simulink model "wednesday_stuff"  (R2022b)
settings: Solver=FixedStepAuto  StartTime=0.0  StopTime=Inf  RelTol=1e-3  EnableMultiTasking=on
values from neighbouring files (symbols this model uses):
  A = [A_sub-k_c.*Bd_sub*C_sub, k_c.*Bd_sub*C_sub; k_c.*Bd_sub2*C_sub, A_sub2-k_c.*Bd_sub2*C_sub]    [doubpend.m]
  b = 0    [doubpend.m]
  J_pend = J_rotor    (= 1.911e-05)    [doubpend.m]
  K_g = m*g*l_c    (= 0.00896720076)    [doubpend.m]
  K_m = 3.9e-2    (= 0.039)    [doubpend.m]
  K_pend = 0    [doubpend.m]
  K_SF = K_aug(1:size(A_d,1))    [doubpend.m]
  K_sin = cos(Angle_Pendu)    [doubpend.m]
  L = 0.23e-3    (= 0.00023)    [doubpend.m]
  L_Pred = L_Pred'    [doubpend.m]
  N = 1/freqresp(TF_yrf,[0])    [doubpend.m]
  R = 8.985    [doubpend.m]
  Stepsize = 1    [doubpend.m]
  Ts = 0.001    [doubpend.m]
  V_s = 10.72    [doubpend.m]
undefined symbols (not defined in the file or in its folder): A_d, B_d, C_d, Down, GPTRIP1SEL, GPTRIP2SEL, TZ1, TZ2, Up
libraries: tiiqmathlib x4, c2837xDlib x1, simulink x1, embmathops x1, c2802xlib x1, c280xlib x1
settings Model: ExtModeTrigDuration=8  Creator=hanw  LastModifiedBy=pruth
settings SolverCC: AutoInsertRateTranBlk=on
settings DataIOCC: InspectSignalLogs=on
settings OptimizationCC: DefaultUnderspecifiedDataType=single  EnhancedBackFolding=on  PassReuseOutputArgsAs=Individual arguments  MaxStackSize=1024  OptimizeBlockOrder=speed  DifferentSizesBufferReuse=on  OptimizationCustomize=off  DenormalBehavior=FlushToZero  EfficientTunableParamExpr=on
settings DebuggingCC: ParameterTunabilityLossMsg=error
settings HardwareCC: ProdBitPerChar=16  ProdBitPerInt=16  ProdBitPerPointer=32  ProdBitPerSizeT=32  ProdBitPerPtrDiffT=32  ProdLargestAtomicInteger=Integer  ProdLargestAtomicFloat=None  ProdWordSize=16  ProdLongLongMode=on  ProdHWDeviceType=Texas Instruments->C2000
settings ModelReferenceCC: ModelReferenceNumInstancesAllowed=Single
settings SFSimCC: MATLABDynamicMemAlloc=off
settings RTWCC: Description=Embedded Coder  SystemTargetFile=ert.tlc  HardwareBoard=TI Delfino F28379D LaunchPad  TLCOptions=-aInlineSetEventsForThisBaseRateFcn=TLC_FALSE -aSuppressMultiTaskScheduler=TLC_FALSE -aRateBasedStepFcn=1  TemplateMakefile=ert_default_tmf  Toolchain=Texas Instruments Code Composer Studio (C2000)
settings CodeAppCC: ForceParamTrailComments=on  IgnoreCustomStorageClasses=off  OperatorAnnotations=on  SimulinkDataObjDesc=on  SFDataObjDesc=on  InsertBlockDesc=on
settings ERTTargetCC: CodeReplacementLibrary=TI C28x  ExtModeTransport=4  ExtModeStaticAlloc=on  ExtModeMexFile=ext_xcp  ExtModeIntrfLevel=Level2 - Open

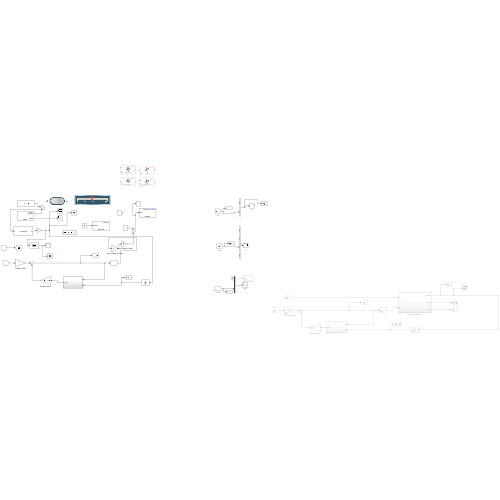
[thumbnail: Simulink's stored preview of the top-level diagram]
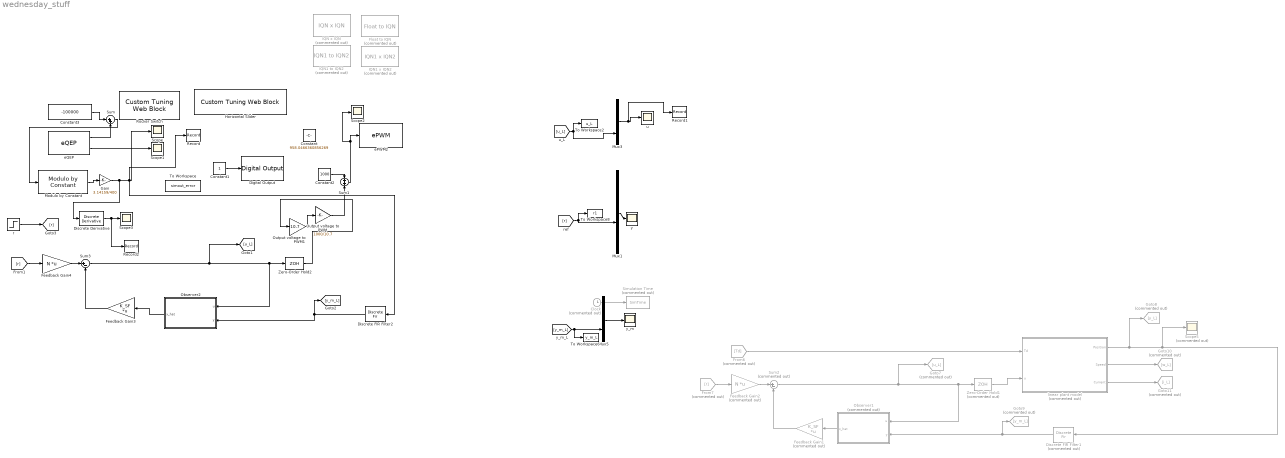
== system wednesday_stuff ==
  Clock : Clock  Commented=on
  Constant : Constant  Value=958.0466360856269
  Constant1 : Constant
  Constant2 : Constant  Value=1000
  Constant3 : Constant  Value=-100000
  Digital Output : c2837xDlib/Digital Output  GPIO_Number=GPIO0~GPIO7  GPIO_Bit0=off  GPIO_BIT0_Toggle=off  GPIO_Bit1=off  GPIO_BIT1_Toggle=off  GPIO_Bit2=on  GPIO_BIT2_Toggle=off  GPIO_Bit3=off  GPIO_BIT3_Toggle=off  GPIO_Bit4=off  GPIO_BIT4_Toggle=off  GPIO_Bit5=off  GPIO_BIT5_Toggle=off  GPIO_Bit6=off  GPIO_BIT6_Toggle=off  GPIO_Bit7=off  GPIO_BIT7_Toggle=off
  Discrete Derivative : simulink/Discrete/Discrete Derivative  gainval=1.0  ICPrevScaledInput=0.0  OutMin=[]  OutMax=[]  OutDataType=fixdt(1, 16)  OutScaling=2^-10  DoSatur=off
  Discrete FIR Filter1 : DiscreteFir  Commented=on  Coefficients=[1]  SampleTime=Ts
  Discrete FIR Filter2 : DiscreteFir  Coefficients=[1]  SampleTime=Ts
  Feedback Gain1 : Gain  Commented=on  Gain=K_SF  Multiplication=Matrix(K*u)
  Feedback Gain2 : Gain  Commented=on  Gain=N  Multiplication=Matrix(K*u)
  Feedback Gain3 : Gain  Gain=K_SF  Multiplication=Matrix(K*u)
  Feedback Gain4 : Gain  Gain=N  Multiplication=Matrix(K*u)
  Float to IQN : tiiqmathlib/Float to IQN  Commented=on  Q_value=10
  From6 : From  Commented=on  GotoTag=Td
  From7 : From  Commented=on  GotoTag=r
  Gain : Gain  Gain=3.14159/400
  Goto10 : Goto  Commented=on  GotoTag=w_L
  Goto11 : Goto  Commented=on  GotoTag=i_L
  Goto7 : Goto  Commented=on  GotoTag=u_L
  Goto8 : Goto  Commented=on  GotoTag=y_L
  Goto9 : Goto  Commented=on  GotoTag=y_m_L
  Horizontal Slider : CustomTuningWebBlock  LabelPosition=Hide  ShowInitialText=on  Configuration="{\"components\":[{\"name\":\"LinearScaleComponent\",\"settings\":{\"bounds\":{\"max\":2000,\"min\":0,\"tickInterval\":\"auto\"},\"internalTickHeightScaleFactor\":0.5,\"labelColor\":[255,255,200],\"labelFont\":{\"font\":\"Arial\",\"fontSize\":12},\"labelOffset\":0.05,\"labelTransparency\":1,\"needleImage\":{\"size\":[596,842],\"src\":\"data:image\\/svg+xml;base64,PD94bWwgdmVyc2lvbj0iMS4wIiBlbmNvZGluZz0idXRmLTgiPz4NCjwhLS0gR2VuZXJhdG9yOiBBZG9iZSBJbGx1c3RyYXRvciAyNS4wLjAsIFNWRyBFeHBvcnQgUGx1Zy1JbiAuIFNWRyBWZXJzaW9uOiA2LjAwIEJ1aWxkIDApICAtLT4NCjxzdmcgdmVyc2lvbj0iMS4xIg0KCSBpZD0ic3ZnOCIgeG1sbnM6Y2M9Imh0dHA6Ly9jcmVhdGl2ZWNvbW1vbnMub3JnL25zIyIgeG1sbnM6ZGM9Imh0dHA6Ly9wdXJsLm9yZy9kYy9lbGVtZW50cy8xLjEvIiB4bWxuczppbmtzY2FwZT0iaHR0cDovL3d3dy5pbmtzY2FwZS5vcmcvbmFtZXNw ...(+2420 chars)\",\"srcOrientation\":\"Right\"},\"needleOffset\":[-0.8044596912521441,-0.0642123287671233],\"needleSize\":{\"height\":0.4337797619047619,\"width\":0.07668067226890757},\"position\":[0.2829861111111111,0.04398634453781513,0.9196428571428571,0.6088789682539683],\"referencePoint\":\"auto\",\"scaleColors\":[],\"scaleColorsSize\":0.2,\"scaleDirection\":\"LR\",\"showLabels\":1,\"showMinorTicks\":0,\"showSpanLine\":1,\"showTicks\":1,\"tickColor\":[252,252,197],\"tickTransparency\":1,\"valueBarColor\":[0,114,189],\"valueBarOffset\":-0.27,\"valueBarSize\":0.1,\"valueBarTransparency\":1}},{\"name\":\"BackgroundImageComponent\",\"settings\":{\"image\":{\"size\":[380,101],\"src\":\"data:image\\/svg+xml;base64,PHN2ZyB4bWxucz0iaHR0cDovL3d3dy53My5vcmcvMjAwMC9zdmciIHhtbG5zOnhsaW5rPSJodHRwOi8vd3d3LnczLm9yZy8xOTk5L3hsaW5rIiB2aWV3Qm94PSIwIDAgMzgwIDEwMSI+PGRlZnM+PHN0eWxlPi5jbHMtMXtmaWxsOiMwMDJiNDI7fS5jbHMtMntmaWxsOiM0MjcwODI7fS5jbHMtM3tmaWxsOnVybCgjcmFkaWFsLWdyYWRpZW50KTt9LmNscy00e2ZpbGw6I2M4YzhjODtzdHJva2U6IzAwMDt9PC9zdHlsZT48cmFkaWFsR3JhZGllbnQgaWQ9InJhZGlhbC1ncmFkaWVudCIgY3g9IjE5MCIgY3k9IjUwLjUiIHI9IjI2OS4yMSIgZ3JhZGllbnRVbml0cz0idXNlclNwYWNlT25Vc2UiPjxzdG9wIG9mZnNldD0iMC4wMSIgc3RvcC1jb2xvcj0iIzNlNGY1OCIvPjxzdG9wIG9mZnNldD0iMC4wNiIgc3RvcC1jb2xvcj0iIzQ0NTc2MSIvPjxzdG9wIG9mZnNldD0iMC4xNSIgc3RvcC1jb2xvcj0iIzU1NmE3NiIvPjxzdG9wIG9mZnNldD0iMC4yNSIgc3RvcC1jb2xvcj0iIzZkODg5NSIvPjxzdG9wIG9mZnNldD0iMC4zOCIgc3RvcC1jb2xvcj0iIzhmYjJjMyIvPjxzdG9wIG9mZnNldD0iMC41MiIgc3RvcC1jb2xvcj0iI2I2ZTRmYSIvPjxzdG9wIG9mZnNldD0iMSIgc3RvcC1jb2xvcj0iIzE1NDY1NyIvPjwvcmFkaWFsR3JhZGllbnQ+PC9kZWZzPjxnIGlkPSJmcmFtZSI+PGcgaWQ9IkxheWVyXzIiIGRhdGEtbmFtZT0iTGF5ZXIgMiI+PGcgaWQ9IkxheWVyXzEtMiIgZGF0YS1uYW1lPSJMYXllciAxLTIiPjxyZWN0IGlkPSJyZWN0MTAzNiIgY2xhc3M9ImNscy0xIiB4PSIxMSIgeT0iMTEiIHdpZHRoPSIzNTgiIGhlaWdodD0iNzkiLz48cGF0aCBpZD0icGF0aDEwMzgiIGNsYXNzPSJjbHMtMiIgZD0iTTgsOFY5M0gzNzJWOFpNMzY5LDkwSDExVjExSDM2OVoiLz48cGF0aCBpZD0icGF0aDEwNDAiIGNsYXNzPSJjbHMtMyIgZD0iTTAsMFYxMDFIMzgwVjBaTTM3Miw5M0g4VjhIMzcyWiIvPjwvZz48L2c+PC9nPjxnIGlkPSJ0cmFjayI+PHBhdGggaWQ9InJlY3QxNjExIiBjbGFzcz0iY2xzLTQiIGQ9Ik0zMy4zNywyNi41OUgzNDYuNjNjNCwwLDcuMjUsMi42LDcuMjUsNS44MWgwYzAsMy4yMS0zLjI1LDUuODItNy4yNSw1LjgySDMzLjM3Yy00LDAtNy4yNS0yLjYxLTcuMjUtNS44MmgwQzI2LjEyLDI5LjE5LDI5LjM3LDI2LjU5LDMzLjM3LDI2LjU5WiIvPjwvZz48L3N2Zz4=\",\"srcOrientation\":\"horizontal\"},\"position\":[0,0,1,1],\"scaleMode\":\"0\"}},{\"name\":\"ForegroundImageComponent\",\"settings\":{\"image\":{\"size\":[0,0],\"src\":\"default\",\"srcOrientation\":[]},\"isForeground\":1,\"position\":[0,0,1,1],\"scaleMode\":\"0\"}}],\"settings\":{\"BindingType\":\"param\",\"aspectRatio\":3.7777777777777777,\"backgroundColor\":[0,0,0,\"1\"],\"backgroundOffset\":0,\"backgroundOpacity\":1,\"fixedAspectRatio\":\"on\",\"foregroundColor\":[252,252,196],\"orientation\":\"horizontal\",\"showBackgroundColor\":false,\"value\":0,\"version\":\"R2022b\"},\"type\":\"LinearGauge\"}"
  IQN x IQN : tiiqmathlib/IQN x IQN  Commented=on  multiplyOption=Multiply
  IQN1 to IQN2 : tiiqmathlib/IQN1 to IQN2  Commented=on  New_Q=10
  IQN1 x IQN2 : tiiqmathlib/IQN1 x IQN2  Commented=on  Q=10
  Modulo by Constant : embmathops/Modulo by Constant  Denominator=400  SimulateUsing=Code generation
      settings: LibrarySourceBlock=embeddedMathLib/Modulo by Constant
  Mux1 : Mux
  Mux3 : Mux  Inputs=2
  Mux5 : Mux  Inputs=2
  Observer1 : Subsystem  Commented=on
  Observer2 : Subsystem
  Output voltage to PWM : Gain  Gain=1000/10.7
  Output voltage to PWM1 : Gain  Gain=10.7
  Record : Record  FileSettingsInternal="{\"entries\":[{\"content\":{\"excelSettings\":{\"content\":{},\"type\":\"Streamout.ExcelSettings\"}},\"type\":\"Streamout.FileSettingStorage\",\"uuid\":\"4d44a113-255c-4606-b9fa-687f08685d0f\"}],\"packageUris\":[\"http://schema.mathworks.com/mf0/streamout_blocks/R2020a\"],\"version\":\"1.0\"}"  SignalsInternal="{\"entries\":[{\"content\":{\"signals\":[{\"content\":{\"blockPath\":[\"wednesday_stuff/Record\"],\"channel\":[],\"dimensions\":[1,1],\"domain\":\"wednesday_stuff/Record\",\"lineColor\":\"#64d413\",\"plots\":[1],\"port\":1,\"sid\":[],\"signalID\":19992,\"signalName\":\"Gain\"},\"type\":\"RecordBlkView.Signal\",\"uuid\":\"3b113f77-257b-44e4-b3fb-c5bb5a30da61\"}]},\"type\":\"RecordBlkView.InputSignals\",\"uuid\":\"18fdf491-a986-43b1-906f-4e09ae16b740\"}],\"packageUris\":[\"http://schema.mathworks.com/mf0/streamout_blocks/R2020a\"],\"version\":\"1.0\"}"  VisualizationBindings="{\"sparklinesplugin\":{\"info\":[{\"bindingParametersList\":[],\"subplotID\":1}]}}"
  Record1 : Record  FileSettingsInternal="{\"entries\":[{\"content\":{\"excelSettings\":{\"content\":{},\"type\":\"Streamout.ExcelSettings\"}},\"type\":\"Streamout.FileSettingStorage\",\"uuid\":\"0aac1b3e-fee5-4f5d-83b4-dff1f84cc0c0\"}],\"packageUris\":[\"http://schema.mathworks.com/mf0/streamout_blocks/R2020a\"],\"version\":\"1.0\"}"  SignalsInternal="{\"entries\":[{\"content\":{\"signals\":[{\"content\":{\"blockPath\":[\"wednesday_stuff/Record1\"],\"channel\":[],\"dimensions\":[2],\"domain\":\"wednesday_stuff/Record1\",\"hasChildren\":true,\"lineColor\":\"#d95319\",\"plots\":[],\"port\":1,\"sid\":[],\"signalID\":19983,\"signalName\":\"Mux3\"},\"type\":\"RecordBlkView.Signal\",\"uuid\":\"6e082fb6-09ee-4524-a44a-0b124cfc634e\"},{\"content\":{\"blockPath\":[\"wednesday_stuff/Record1\"],\"channel\":[1],\"dimensions\":[2],\"domain\":\"wednesday_stuff/Record1\",\"lineColor\":\"#a2142f\",\"parentID\":19983,\"plots\":[1],\"port\":1,\"sid\":[],\"signalID\":19984,\"signalName\":\"Mux3\"},\"type\":\"RecordBlkView.Signal\",\"uuid\":\"8481b1b3-e8f1-429e-8ea8-884c20c8de04\"},{\"content\":{\"blockPath\":[\"wednesday_stuff/Record1\"],\"channel\":[2],\"dimensions\":[2],\"domain\":\"wednesday_stuff/Record1\",\"lineColor\":\"#ff6929\",\"parentID\":19983,\"plots\":[1],\"port\":1,\"sid\":[],\"signalID\":19985,\"signalName\":\"Mux3\"},\"type\":\"RecordBlkView.Signal\",\"uuid\":\"e82f2203-a385-483f-b916-afcb370bf19b\"}]},\"type\":\"RecordBlkView.InputSignals\",\"uuid\":\"b3968912-3d6b-4861-86d9-c36083a10435\"}],\"packageUris\":[\"http://schema.mathworks.com/mf0/streamout_blocks/R2020a\"],\"version\":\"1.0\"}"  VisualizationBindings="{\"sparklinesplugin\":{\"info\":[{\"bindingParametersList\":[],\"subplotID\":1}]}}"
  Record2 : Record  FileSettingsInternal="{\"entries\":[{\"content\":{\"excelSettings\":{\"content\":{},\"type\":\"Streamout.ExcelSettings\"}},\"type\":\"Streamout.FileSettingStorage\",\"uuid\":\"185a5fe7-9dc5-4829-8d1e-3b701eb1b41e\"}],\"packageUris\":[\"http://schema.mathworks.com/mf0/streamout_blocks/R2020a\"],\"version\":\"1.0\"}"  SignalsInternal="{\"entries\":[{\"content\":{\"signals\":[{\"content\":{\"blockPath\":[\"wednesday_stuff/Record2\"],\"channel\":[],\"dimensions\":[1,1],\"domain\":\"wednesday_stuff/Record2\",\"lineColor\":\"#77ac30\",\"plots\":[1],\"port\":1,\"sid\":[],\"signalID\":19978,\"signalName\":\"Discrete Derivative\"},\"type\":\"RecordBlkView.Signal\",\"uuid\":\"3faa6981-de14-4794-b670-d27a9092c6dd\"}]},\"type\":\"RecordBlkView.InputSignals\",\"uuid\":\"b823a2af-b6b8-4942-aa66-d3cc61a8ed73\"}],\"packageUris\":[\"http://schema.mathworks.com/mf0/streamout_blocks/R2020a\"],\"version\":\"1.0\"}"  VisualizationBindings="{\"sparklinesplugin\":{\"info\":[{\"bindingParametersList\":[],\"subplotID\":1}]}}"
  Rocker Switch : CustomTuningWebBlock  LabelPosition=Hide  ShowInitialText=on  Configuration="{\"components\":[{\"name\":\"CustomSwitchStateComponent\",\"settings\":{\"position\":[0,0,1,1],\"states\":[{\"HitRegion\":{\"position\":[0,0,0.5,1]},\"Image\":{\"position\":[0.13,0,1,0.75],\"size\":[1,0.75],\"src\":\"data:image\\/svg+xml;base64,PHN2ZyB4bWxucz0iaHR0cDovL3d3dy53My5vcmcvMjAwMC9zdmciIHhtbG5zOnhsaW5rPSJodHRwOi8vd3d3LnczLm9yZy8xOTk5L3hsaW5rIiB2aWV3Qm94PSIwIDAgNzUgMjQuOCI+PGRlZnM+PHN0eWxlPi5jbHMtMXtmaWxsOnVybCgjcmFkaWFsLWdyYWRpZW50KTt9LmNscy0ye2ZpbGw6dXJsKCNyYWRpYWwtZ3JhZGllbnQtMik7fS5jbHMtM3tzdHJva2U6I2IyMDAwMDtzdHJva2Utd2lkdGg6MC4yNXB4O2ZpbGw6dXJsKCNsaW5lYXItZ3JhZGllbnQpO30uY2xzLTR7ZmlsbDp1cmwoI2xpbmVhci1ncmFkaWVudC0yKTt9LmNs ...(+3576 chars)\",\"srcOrientation\":\"Right\"},\"Label\":{\"color\":[0.5019607843137255,0.5019607843137255,0.5019607843137255],\"icon\":{\"size\":[0,0],\"src\":[],\"srcOrientation\":\"Right\"},\"iconPlacement\":\"left\",\"opacity\":1,\"position\":[0.5,0.08],\"show\":true,\"text\":{\"content\":\"Off\",\"font\":\"Helvetica\",\"fontSize\":29.7154725}},\"Value\":0},{\"HitRegion\":{\"position\":[0,0.5,0.5,1]},\"Image\":{\"position\":[0.13,0,1,0.75],\"size\":[1,0.75],\"src\":\"data:image\\/svg+xml;base64,PHN2ZyB4bWxucz0iaHR0cDovL3d3dy53My5vcmcvMjAwMC9zdmciIHhtbG5zOnhsaW5rPSJodHRwOi8vd3d3LnczLm9yZy8xOTk5L3hsaW5rIiB2aWV3Qm94PSIwIDAgNzUgMjQuOCI+PGRlZnM+PHN0eWxlPi5jbHMtMXtmaWxsOnVybCgjcmFkaWFsLWdyYWRpZW50KTt9LmNscy0ye2ZpbGw6dXJsKCNyYWRpYWwtZ3JhZGllbnQtMik7fS5jbHMtM3tzdHJva2U6I2IyMDAwMDtzdHJva2Utd2lkdGg6MC4yNXB4O2ZpbGw6dXJsKCNsaW5lYXItZ3JhZGllbnQpO30uY2xzLTR7ZmlsbDp1cmwoI2xpbmVhci1ncmFkaWVudC0yKTt9LmNs ...(+3520 chars)\",\"srcOrientation\":\"Right\"},\"Label\":{\"color\":[0.5019607843137255,0.5019607843137255,0.5019607843137255],\"icon\":{\"size\":[0,0],\"src\":[],\"srcOrientation\":\"Right\"},\"iconPlacement\":\"left\",\"opacity\":1,\"position\":[0.5,0.92],\"show\":true,\"text\":{\"content\":\"On\",\"font\":\"Helvetica\",\"fontSize\":29.7154725}},\"Value\":1}]}},{\"name\":\"BackgroundImageComponent\",\"settings\":{\"image\":{\"size\":[155,70],\"src\":\"default\",\"srcOrientation\":\"Right\"},\"position\":[0,0,1,1],\"scaleMode\":\"0\"}},{\"name\":\"ForegroundImageComponent\",\"settings\":{\"image\":{\"size\":[0,0],\"src\":\"default\",\"srcOrientation\":[]},\"isForeground\":1,\"position\":[0,0,1,1],\"scaleMode\":\"0\"}}],\"settings\":{\"BindingType\":\"param\",\"backgroundColor\":[0,0,255,\"1\"],\"backgroundOffset\":0.14,\"fixedAspectRatio\":\"on\",\"foregroundColor\":[234,234,234],\"showBackgroundColor\":false,\"variant\":\"rocker\",\"version\":\"R2022b\"},\"type\":\"Switch\"}"
  Scope{,1..3} (4 alike) : Scope
  Scope5 : Scope  Commented=on
  Simulation Time : ToWorkspace  Commented=on  VariableName=SimTime  SampleTime=-1
  Sum : Sum  Inputs=|++
  Sum1 : Sum
  Sum2 : Sum  Commented=on  Inputs=|+-
  Sum3 : Sum  Inputs=|+-
  To Workspace : ToWorkspace  VariableName=simout_error  SaveFormat=Timeseries  SampleTime=-1
  To Workspace2 : ToWorkspace  VariableName=u_L  SampleTime=Ts
  To Workspace6 : ToWorkspace  VariableName=y_m_L  SampleTime=Ts
  To Workspace8 : ToWorkspace  VariableName=r1  SampleTime=Ts
  Zero-Order Hold1 : ZeroOrderHold  Commented=on  SampleTime=Ts
  Zero-Order Hold2 : ZeroOrderHold  SampleTime=Ts
  ePWM2 : c2802xlib/ePWM  PwmType=C2000_Type4  useModule=ePWM1  ePWMxLINKTBPRD=Not Linked  periodUnits=Clock cycles  timerSource=Specify via dialog  timerPeriod_clk=2000  timerPeriod_sec=0.0001  tbshadow=Counter equals to zero  countingMode=Up-Down  phaseActiveEnable=Disable  phaseDirection=Count down after sync  phaseActive=0  synchronizationEnable=off  dcaevt1Sync=off  dcbevt1Sync=off  synchronizationOption=Counter equals to zero (CTR=Zero)  dcbevt1SyncOut=off  dcaevt1SyncOut=off  cmpdSyncOut=off  cmpcSyncOut=off  cmpbSyncOut=off  zeroSyncOut=on  swfSyncOut=off  perSynchronizationOption=Counter equals to period (CTR=PRD)  clockPrescale=1  HSclockPrescale=1  enswap=off  ePWMxAStatus=on  ePWMxAactionLogic1=Do nothing  ePWMxAactionLogic2=Do nothing  ePWMxAactionLogic3=Clear  ePWMxAactionLogic4=Set  ePWMxAactionLogic5=Do nothing  ePWMxAactionLogic6=Do nothing  ePWMxACSFenable=off  ePWMxACSFvalue=Forcing disable  ePWMxASFreload=Zero  ePWMxBStatus=on  ePWMxBactionLogic1=Set  ePWMxBactionLogic2=Clear  ePWMxBactionLogic3=Do nothing  ePWMxBactionLogic4=Do nothing  ePWMxBactionLogic5=Clear  ePWMxBactionLogic6=Set  ePWMxBCSFenable=off  ePWMxBCSFvalue=Forcing disable  ePWMxBSFreload=Zero  ePWNxBOutWay=off  ePWMxLINKCMPA=Not Linked  CMPAUnits=Clock cycles  CMPASource=Input port  CMPAValue_per=50  CMPAValue_clk=floor(2000/2+1)  enCMPAshadow=Counter equals to zero (CTR=Zero)  ePWMxLINKCMPB=Not Linked  CMPBUnits=Clock cycles  CMPBSource=Specify via dialog  CMPBValue_per=50  CMPBValue_clk=floor(2000/2+1)  enCMPBshadow=Counter equals to zero (CTR=Zero)  ePWMxLINKCMPC=ePWM3  CMPCUnits=Clock cycles  CMPCSource=Specify via dialog  CMPCValue_per=50  CMPCValue_clk=32000  enCMPCshadow=Counter equals to zero (CTR=Zero)  ePWMxLINKCMPD=Not Linked  CMPDUnits=Clock cycles  CMPDSource=Specify via dialog  CMPDValue_per=50  CMPDValue_clk=1000  enCMPDshadow=Counter equals to zero (CTR=Zero)  enableDBePWMxA=on  enableDBePWMxB=on  enhalfcycle=off  DBpolarity=Active high complementary (AHC)  DBedgeDelay=Positive  DBSource_ePWMxA=ePWMxA  DBSource_ePWMxB=ePWMxA  DBPeriodUnits=Clock cycles  DBperiodSource=Specify via dialog  REDperiod=15  FEDperiod=15  REDperiod_sec=0  FEDperiod_sec=0  LoadModeDBRED=Immediate without using shadow  LoadModeDBFED=Immediate without using shadow  adcstartModuleA=on  adcrequestEventA=First event  adcstartEventA=Digital Compare Module A Event 1 start of conversion (DCAEVT1.soc)  adcstartEventA_type2=Counter equals to period (CTR=PRD)  adcstartModuleB=off  adcrequestEventB=First event  adcstartEventB=Counter equals to zero (CTR=Zero)  adcstartEventB_type2=Counter equals to zero (CTR=Zero)  intEn=off  intPrd=First event  intSel=Counter equals to zero (CTR=Zero)  intSel_type2=Counter equals to zero (CTR=Zero)  hrpe=off  enHRPWM=off  HRPWM_LoadMode=Counter equals to period (CTR=PRD)  HRPWM_CTLMode=Duty or Period control mode  HRPWM_EDGMode=Both edge  hrpeb=off  enHRPWMB=off  HRPWM_LoadModeB=Counter equals to zero (CTR=ZERO)  HRPWM_CTLModeB=Duty or Period control mode  HRPWM_EDGModeB=Both edge  enHRDBRED=off  enHRDBFED=off  enSFO=on  enautoconv=on  chopperEnable=off  chopperFrequency=1  chopperFirstwidth=1  chopperDuty=12.5%  tripZonesource=Specify via dialog  tzselOSHT1=off  tzselOSHT2=off  tzselOSHT3=off  tzselOSHDCAEV1=off  tzselOSHDCBEV1=off  tzselCBC1=off  tzselCBC2=off  tzselCBC3=off  tzselCBCDCAEV2=off  tzselCBCDCBEV2=off  tzselOSHT4=off  tzselOSHT5=off  tzselOSHT6=off  tzselCBC4=off  tzselCBC5=off  tzselCBC6=off  enTzOstIntr=off  enTzCbcIntr=off  enTzDCAEVT1Intr=off  enTzDCAEVT2Intr=off  enTzDCBEVT1Intr=off  enTzDCBEVT2Intr=off  ePWMxAforced=No action  ePWMxBforced=No action  DCAEVT1forced=No action  DCBEVT1forced=No action  DCAEVT2forced=No action  DCBEVT2forced=No action  dcah=Trip Zone 1 input (TZ1)  dcal=Trip Zone 2 input (TZ2)  dcbh=Trip Zone 1 input (TZ1)  dcbl=Trip Zone 2 input (TZ2)  dcah_type2=GPTRIP1SEL/(TZ1)  dcal_type2=GPTRIP2SEL/(TZ2)  dcbh_type2=GPTRIP1SEL/(TZ1)  dcbl_type2=GPTRIP2SEL/(TZ2)  gendcaevt1=Event disabled  gendcaevt2=Event disabled  gendcbevt1=Event disabled  gendcbevt2=Event disabled  dcaevt1src=DCAEVT1 with sync  dcaevt2src=DCAEVT2 with sync  dcbevt1src=DCBEVT1 with sync  dcbevt2src=DCBEVT2 with sync  pulsesel=Counter equals to zero (CTR=Zero)  blankinv=off  blankoffset=0  blankwidth=0  evsrcsel=Filtered version of DCAEVT1 (DCAEVT1FILT)  encape=off
  eQEP : c280xlib/eQEP  useModule=eQEP1  pcInputmode=Quadrature-count  externalClockrate=2x resolution: Count the rising/falling edge  swapPolarityselection=Clockwise  qdfOutputport=off  qapPolarityselection=off  qbpPolarityselection=off  qipPolarityselection=off  qspPolarityselection=off  igatePolarityselection=off  sampleTime=0.001  pcOutputport=on  pcMaximumvalue=4294967295  indexInitializationcheck=off  indexInitializationevent=Rising edge  strobeInitializationcheck=off  strobeInitializationevent=Rising edge  softwareInitializationcheck=on  softwareInitializationsource=Set to init value at start up  softwareInitializationmode=on  pcInitialvalue=100000  pcResetmode=Reset on the maximum position  ieloutputport=off  indexEventlatch=Rising edge  seloutputport=off  strobeEventlatch=Rising edge  pcefOutputport=off  enableEqepcapture=on  qctmrOutputport=off  qcprdOutputport=on  captureTimerprescaler=64  upEventprescaler=1  overflowErrorflag=off  directionErrorflag=off  captureTimerposition=On position counter read  unitTimerperiod=100000000  captureTimerlatch=off  capturePeriodlatch=off  positionCounterlatch=off  soenPolarityselection=off  spselPolarityselection=Index pin is used for sync output  compareValuesource=Specify via dialog  shadowMode=Load on QPOSCNT=0  compareValue=4294967295  syncOutputwidth=1  polaritySyncoutput=Active high  watchdogEnable=off  watchdogTimer=65535  outport1Datatype=auto  outport2Datatype=auto  outport3Datatype=auto  outport4Datatype=auto  outport5Datatype=auto  outport6Datatype=auto  outport7Datatype=auto  outport8Datatype=auto  outport9Datatype=auto  outport10Datatype=auto  outport11Datatype=auto  outport12Datatype=auto  eqepinterrupt_pce=off  eqepinterrupt_qpe=off  eqepinterrupt_qdc=off  eqepinterrupt_wto=off  eqepinterrupt_pcu=off  eqepinterrupt_pco=off  eqepinterrupt_pcr=off  eqepinterrupt_pcm=off  eqepinterrupt_sel=off  eqepinterrupt_iel=off  eqepinterrupt_uto=off  pheOutputport=off  watchdogOutputport=off  outport13Datatype=auto  outport14Datatype=auto
  linear plant model : Subsystem  Commented=on
  r : Step  After=Stepsize  SampleTime=Ts
  u : Scope
  y : Scope
  y_m : Scope
  wires:
  Constant1/1 -> Digital Output/1
  Output voltage to PWM/1 -> Sum1/2
  Constant2/1 -> Sum1/1
  Sum1/1 -> Scope2/1, ePWM2/1
  eQEP/2 -> Scope1/1
  Output voltage to PWM1/1 -> Output voltage to PWM/1
  Feedback Gain1/1 -> Sum2/2
  Observer1/1(x_hat) -> Feedback Gain1/1
  From6/1 -> linear plant model/1(Td)
  linear plant model/2(Speed) -> Goto10/1
  Clock/1 -> Simulation Time/1
  Discrete FIR Filter1/1 -> Observer1/2(y), Goto9/1
  Zero-Order Hold1/1 -> linear plant model/2(u)
  linear plant model/1(Position) -> Goto8/1, Scope5/1, Discrete FIR Filter1/1
  Feedback Gain2/1 -> Sum2/1
  From7/1 -> Feedback Gain2/1
  Sum2/1 -> Goto7/1, Observer1/1(u), Zero-Order Hold1/1
  linear plant model/3(Current) -> Goto11/1
  Sum3/1 -> [u_L], Observer2/1(u), Zero-Order Hold2/1
  Discrete FIR Filter2/1 -> [y_m_L], Observer2/2(y)
  Zero-Order Hold2/1 -> Output voltage to PWM1/1
  Observer2/1(x_hat) -> Feedback Gain3/1
  [r] -> Feedback Gain4/1
  Feedback Gain3/1 -> Sum3/2
  Feedback Gain4/1 -> Sum3/1
  r/1 -> [r]
  Mux1/1 -> y/1
  [u_L] -> To Workspace2/1, Mux3/2
  [y_m_L] -> To Workspace6/1, Mux5/2
  Mux5/1 -> y_m/1
  [r] -> To Workspace8/1, Mux1/3
  Mux3/1 -> Record1/1, u/1
  Constant3/1 -> Sum/1
  eQEP/1 -> Sum/2
  Modulo by Constant/1 -> Gain/1
  Sum/1 -> Modulo by Constant/1
  Gain/1 -> Discrete Derivative/1, Discrete FIR Filter2/1, Record/1, Scope/1
  Discrete Derivative/1 -> Record2/1, Scope3/1

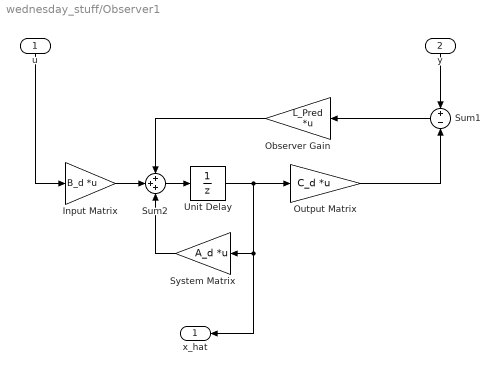
== system wednesday_stuff/Observer1 ==
  u : Inport
  y : Inport  Port=2
  Input Matrix : Gain  Gain=B_d  Multiplication=Matrix(K*u)
  Observer Gain : Gain  Gain=L_Pred  Multiplication=Matrix(K*u)
  Output Matrix : Gain  Gain=C_d  Multiplication=Matrix(K*u)
  Sum1 : Sum  Inputs=+|-
  Sum2 : Sum  Inputs=+++
  System Matrix : Gain  Gain=A_d  Multiplication=Matrix(K*u)
  Unit Delay : UnitDelay  SampleTime=Ts  HasFrameUpgradeWarning=on
  x_hat : Outport
  wires:
  Sum1/1 -> Observer Gain/1
  System Matrix/1 -> Sum2/3
  Sum2/1 -> Unit Delay/1
  Output Matrix/1 -> Sum1/2
  Input Matrix/1 -> Sum2/2
  Observer Gain/1 -> Sum2/1
  u/1 -> Input Matrix/1
  Unit Delay/1 -> x_hat/1, System Matrix/1, Output Matrix/1
  y/1 -> Sum1/1

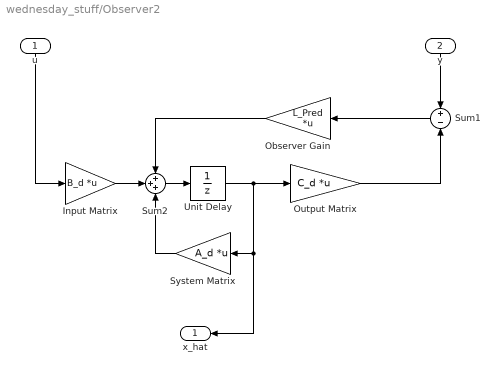
== system wednesday_stuff/Observer2 ==
  u : Inport
  y : Inport  Port=2
  Input Matrix : Gain  Gain=B_d  Multiplication=Matrix(K*u)
  Observer Gain : Gain  Gain=L_Pred  Multiplication=Matrix(K*u)
  Output Matrix : Gain  Gain=C_d  Multiplication=Matrix(K*u)
  Sum1 : Sum  Inputs=+|-
  Sum2 : Sum  Inputs=+++
  System Matrix : Gain  Gain=A_d  Multiplication=Matrix(K*u)
  Unit Delay : UnitDelay  SampleTime=Ts  HasFrameUpgradeWarning=on
  x_hat : Outport
  wires:
  Sum1/1 -> Observer Gain/1
  System Matrix/1 -> Sum2/3
  Sum2/1 -> Unit Delay/1
  Output Matrix/1 -> Sum1/2
  Input Matrix/1 -> Sum2/2
  Observer Gain/1 -> Sum2/1
  u/1 -> Input Matrix/1
  Unit Delay/1 -> x_hat/1, System Matrix/1, Output Matrix/1
  y/1 -> Sum1/1

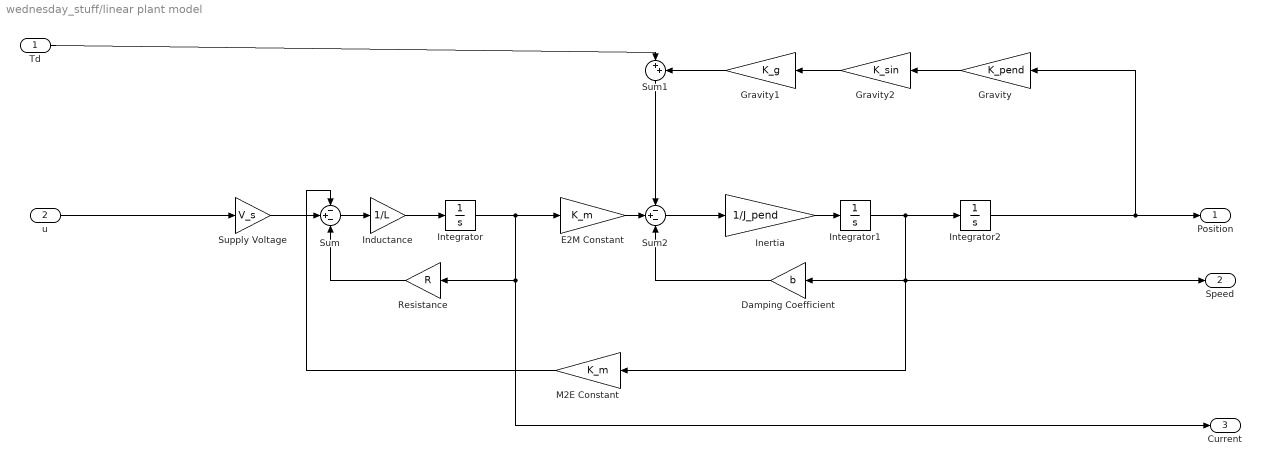
== system wednesday_stuff/linear plant model ==
  Td : Inport
  u : Inport  Port=2
  Damping Coefficient : Gain  Gain=b
  E2M Constant : Gain  Gain=K_m
  Gravity : Gain  Gain=K_pend
  Gravity1 : Gain  Gain=K_g
  Gravity2 : Gain  Gain=K_sin
  Inductance : Gain  Gain=1/L
  Inertia : Gain  Gain=1/J_pend
  Integrator : Integrator
  Integrator1 : Integrator
  Integrator2 : Integrator
  M2E Constant : Gain  Gain=K_m
  Resistance : Gain  Gain=R
  Sum : Sum  Inputs=-+-
  Sum1 : Sum  Inputs=|++
  Sum2 : Sum  Inputs=-+-
  Supply Voltage : Gain  Gain=V_s
  Position : Outport
  Speed : Outport  Port=2
  Current : Outport  Port=3
  wires:
  Damping Coefficient/1 -> Sum2/3
  Sum1/1 -> Sum2/1
  Gravity/1 -> Gravity2/1
  Integrator/1 -> E2M Constant/1, Current/1, Resistance/1
  Integrator1/1 -> Speed/1, M2E Constant/1, Damping Coefficient/1, Integrator2/1
  Resistance/1 -> Sum/3
  Sum/1 -> Inductance/1
  Inductance/1 -> Integrator/1
  Supply Voltage/1 -> Sum/2
  M2E Constant/1 -> Sum/1
  Sum2/1 -> Inertia/1
  Inertia/1 -> Integrator1/1
  E2M Constant/1 -> Sum2/2
  u/1 -> Supply Voltage/1
  Td/1 -> Sum1/1
  Integrator2/1 -> Gravity/1, Position/1
  Gravity1/1 -> Sum1/2
  Gravity2/1 -> Gravity1/1
